simulink model "sistemacompleto"  (Simulink 4.00)
settings: Solver=ode45  StartTime=0.0  StopTime=0.3  MaxStep=0.125e-4  RelTol=1e-3
libraries: simulink3 x2
settings Model: LastModifiedBy=Gui  BooleanDataType=on

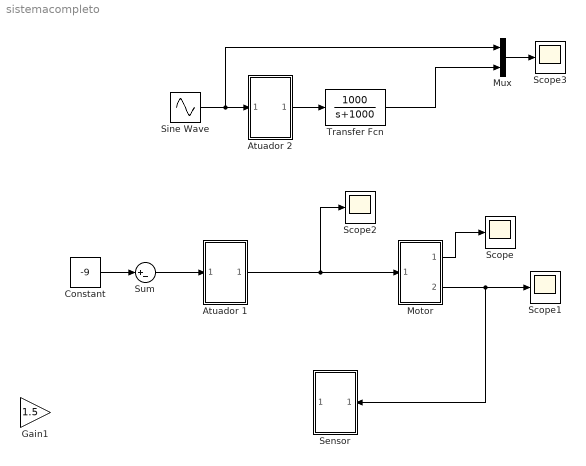
== system sistemacompleto ==
  Atuador 1 : Subsystem
      settings: RTWFcnNameOpts=Auto  RTWFileNameOpts=Auto
  Atuador 2 : Subsystem
      settings: RTWFcnNameOpts=Auto  RTWFileNameOpts=Auto
  Constant : Constant  Value=-9
  Gain1 : Gain  Gain=1.5  Multiplication=Element-wise(K.*u)  SaturateOnIntegerOverflow=on
  Motor : Subsystem
      settings: RTWFcnNameOpts=Auto  RTWFileNameOpts=Auto
  Mux : Mux  Inputs=2
  Scope{,1..3} (4 alike) : Scope
      Scope settings: TimeRange=auto  YMin=-0.3  YMax=1.8  SaveToWorkspace=off  SaveName=ScopeData  MaxDataPoints=5000
      Scope1 settings: TimeRange=auto  YMin=-656.57  YMax=-656.57  SaveToWorkspace=off  MaxDataPoints=5000
      Scope2 settings: TimeRange=auto  YMin=-20  YMax=20  SaveToWorkspace=off  SaveName=ScopeData2  MaxDataPoints=5000
      Scope3 settings: TimeRange=auto  YMin=-3.5  YMax=3.5  SaveToWorkspace=off  SaveName=ScopeData4  MaxDataPoints=5000
  Sensor : Subsystem  Orientation=left
      settings: RTWFcnNameOpts=Auto  RTWFileNameOpts=Auto
  Sine Wave : Sin  SineType=Time-based  Amplitude=1  Bias=0  Frequency=100  Phase=0  Samples=10  SampleTime=0  Offset=0
  Sum : Sum  Inputs=|+-  SaturateOnIntegerOverflow=on
  Transfer Fcn : TransferFcn  Numerator=[1000]  Denominator=[1 1000]  AbsoluteTolerance=auto  Realization=auto
  wires:
  Atuador 1/1(Out1) -> Motor/1(In1), Scope2/1
  Motor/2(Out2) -> Sensor/1(In1), Scope1/1
  Sum/1 -> Atuador 1/1(In1)
  Constant/1 -> Sum/1
  Motor/1(Out1) -> Scope/1
  Sine Wave/1 -> Atuador 2/1(In1), Mux/1
  Atuador 2/1(Out1) -> Transfer Fcn/1
  Mux/1 -> Scope3/1
  Transfer Fcn/1 -> Mux/2

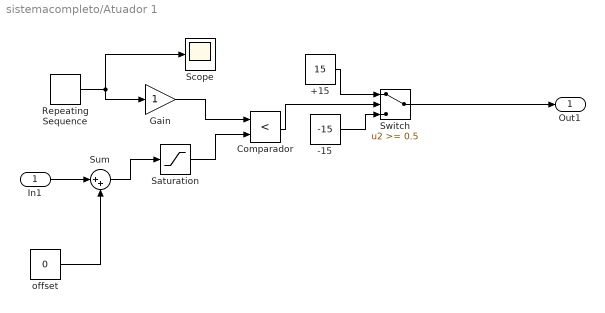
== system sistemacompleto/Atuador 1 ==
  In1 : Inport  Port=1  LatchInput=off
  +15 : Constant  Value=15
  "-15 " : Constant  Value=-15
  Comparador : RelationalOperator  Operator=<
  Gain : Gain  Gain=1  Multiplication=Element-wise(K.*u)  SaturateOnIntegerOverflow=on
  Repeating Sequence : simulink3/Sources/Repeating Sequence  rep_seq_t=[0 1/40000 1/20000]  rep_seq_y=[-5 5 -5]
  Saturation : Saturate  UpperLimit=9  LowerLimit=-9  LinearizeAsGain=on
  Scope : Scope
      settings: TimeRange=auto  YMin=-5  YMax=5  SaveToWorkspace=off  SaveName=ScopeData3  LimitDataPoints=on  MaxDataPoints=5000
  Sum : Sum  Inputs=|++  SaturateOnIntegerOverflow=on
  Switch : Switch  Threshold=0.5
  "offset " : Constant  Value=0
  Out1 : Outport  Port=1
  wires:
  Comparador/1 -> Switch/2
  +15/1 -> Switch/1
  "-15 "/1 -> Switch/3
  Switch/1 -> Out1/1
  In1/1 -> Sum/1
  "offset "/1 -> Sum/2
  Repeating Sequence/1 -> Gain/1, Scope/1
  Gain/1 -> Comparador/1
  Saturation/1 -> Comparador/2
  Sum/1 -> Saturation/1

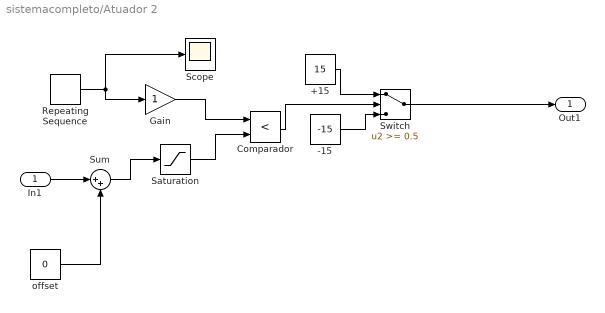
== system sistemacompleto/Atuador 2 ==
  In1 : Inport  Port=1  LatchInput=off
  +15 : Constant  Value=15
  "-15 " : Constant  Value=-15
  Comparador : RelationalOperator  Operator=<
  Gain : Gain  Gain=1  Multiplication=Element-wise(K.*u)  SaturateOnIntegerOverflow=on
  Repeating Sequence : simulink3/Sources/Repeating Sequence  rep_seq_t=[0 1/40000 1/20000]  rep_seq_y=[-5 5 -5]
  Saturation : Saturate  UpperLimit=9  LowerLimit=-9  LinearizeAsGain=on
  Scope : Scope
      settings: TimeRange=auto  YMin=-5  YMax=5  SaveToWorkspace=off  SaveName=ScopeData3  LimitDataPoints=on  MaxDataPoints=5000
  Sum : Sum  Inputs=|++  SaturateOnIntegerOverflow=on
  Switch : Switch  Threshold=0.5
  "offset " : Constant  Value=0
  Out1 : Outport  Port=1
  wires:
  Sum/1 -> Saturation/1
  Saturation/1 -> Comparador/2
  Gain/1 -> Comparador/1
  Repeating Sequence/1 -> Scope/1, Gain/1
  "offset "/1 -> Sum/2
  In1/1 -> Sum/1
  Switch/1 -> Out1/1
  "-15 "/1 -> Switch/3
  +15/1 -> Switch/1
  Comparador/1 -> Switch/2

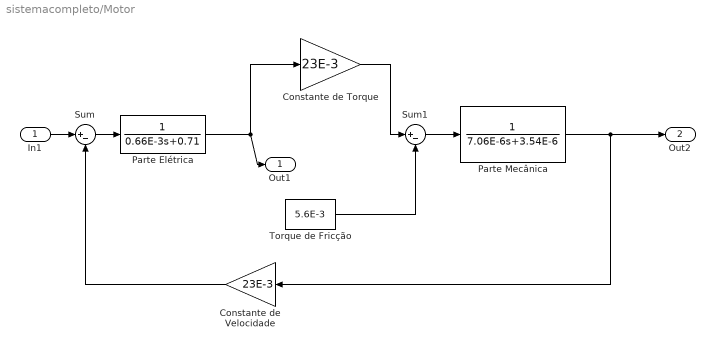
== system sistemacompleto/Motor ==
  In1 : Inport  Port=1  LatchInput=off
  Constante de Torque : Gain  Gain=23E-3  Multiplication=Element-wise(K.*u)  SaturateOnIntegerOverflow=on
  Constante de Velocidade : Gain  Orientation=left  Gain=23E-3  Multiplication=Element-wise(K.*u)  SaturateOnIntegerOverflow=on
  Parte Elétrica : TransferFcn  Numerator=[1]  Denominator=[0.66E-3 0.71]  AbsoluteTolerance=auto  Realization=auto
  Parte Mecânica : TransferFcn  Numerator=[1]  Denominator=[7.06E-6 3.54E-6]  AbsoluteTolerance=auto  Realization=auto
  Sum : Sum  Inputs=|+-  SaturateOnIntegerOverflow=on
  Sum1 : Sum  Inputs=|+-  SaturateOnIntegerOverflow=on
  Torque de Fricção : Constant  Value=5.6E-3
  Out1 : Outport  Port=1
  Out2 : Outport  Port=2
  wires:
  Sum/1 -> Parte Elétrica/1
  Parte Elétrica/1 -> Constante de Torque/1, Out1/1
  Parte Mecânica/1 -> Constante de Velocidade/1, Out2/1
  Constante de Velocidade/1 -> Sum/2
  Constante de Torque/1 -> Sum1/1
  Sum1/1 -> Parte Mecânica/1
  Torque de Fricção/1 -> Sum1/2
  In1/1 -> Sum/1

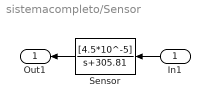
== system sistemacompleto/Sensor ==
  In1 : Inport  Orientation=left  Port=1  LatchInput=off
  "Sensor " : TransferFcn  Orientation=left  Numerator=[4.5*10^-5]  Denominator=[1 305.81]  AbsoluteTolerance=auto  Realization=auto
  Out1 : Outport  Orientation=left  Port=1
  wires:
  "Sensor "/1 -> Out1/1
  In1/1 -> "Sensor "/1
